simulink model "heater_steam_jacket_test"  (R2018b)
settings: Solver=VariableStepAuto  StartTime=0.0  StopTime=10.0  RelTol=1e-3
settings Model: Creator=gv281  LastModifiedBy=gv281

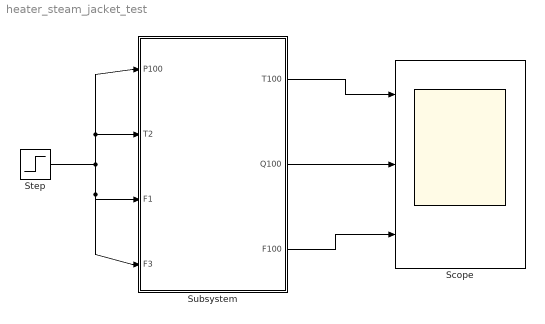
== system heater_steam_jacket_test ==
  Scope : Scope  NumInputPorts=3
  Step : Step  SampleTime=0
  Subsystem : Subsystem
  wires:
  Subsystem/1(T100) -> Scope/1
  Subsystem/3(F100) -> Scope/3
  Subsystem/2(Q100) -> Scope/2
  Step/1 -> Subsystem/3(F1), Subsystem/4(F3), Subsystem/2(T2), Subsystem/1(P100)

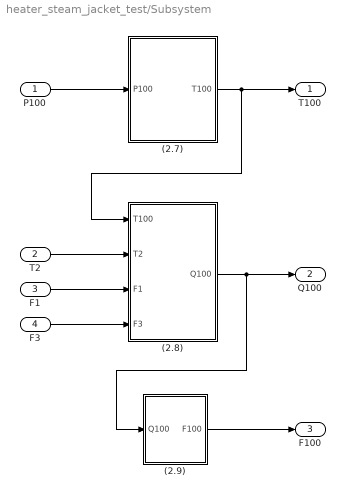
== system heater_steam_jacket_test/Subsystem ==
  P100 : Inport
  T2 : Inport  Port=2
  F1 : Inport  Port=3
  F3 : Inport  Port=4
  (2.7) : Subsystem
  (2.8) : Subsystem
  (2.9) : Subsystem
  T100 : Outport
  Q100 : Outport  Port=2
  F100 : Outport  Port=3
  wires:
  F3/1 -> (2.8)/4(F3)
  (2.9)/1(F100) -> F100/1
  (2.8)/1(Q100) -> Q100/1, (2.9)/1(Q100)
  (2.7)/1(T100) -> T100/1, (2.8)/1(T100)
  P100/1 -> (2.7)/1(P100)
  T2/1 -> (2.8)/2(T2)
  F1/1 -> (2.8)/3(F1)

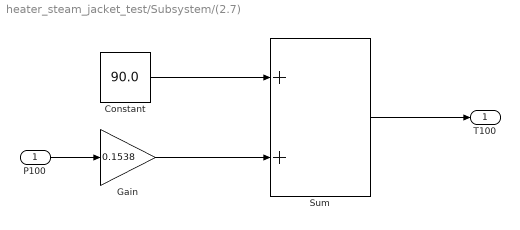
== system heater_steam_jacket_test/Subsystem/(2.7) ==
  P100 : Inport
  Constant : Constant  Value=90.0
  Gain : Gain  Gain=0.1538
  Sum : Sum
  T100 : Outport
  wires:
  Gain/1 -> Sum/2
  P100/1 -> Gain/1
  Constant/1 -> Sum/1
  Sum/1 -> T100/1

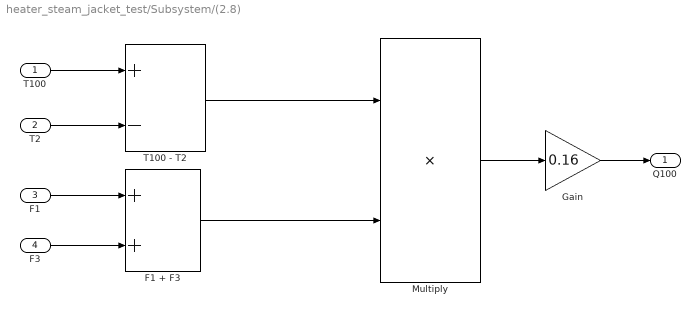
== system heater_steam_jacket_test/Subsystem/(2.8) ==
  T100 : Inport
  T2 : Inport  Port=2
  F1 : Inport  Port=3
  F3 : Inport  Port=4
  F1 + F3 : Sum
  Gain : Gain  Gain=0.16
  Multiply : Product
  T100 - T2 : Sum  Inputs=+-
  Q100 : Outport
  wires:
  Gain/1 -> Q100/1
  T2/1 -> T100 - T2/2
  T100/1 -> T100 - T2/1
  Multiply/1 -> Gain/1
  F1/1 -> F1 + F3/1
  T100 - T2/1 -> Multiply/1
  F1 + F3/1 -> Multiply/2
  F3/1 -> F1 + F3/2

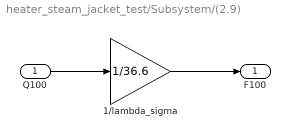
== system heater_steam_jacket_test/Subsystem/(2.9) ==
  Q100 : Inport
  1/lambda_sigma : Gain  Gain=1/36.6
  F100 : Outport
  wires:
  1/lambda_sigma/1 -> F100/1
  Q100/1 -> 1/lambda_sigma/1
